simulink model "Final_Proposal"  (R2024a)
settings: Solver=ode4  StartTime=0.0  StopTime=100  FixedStep=Step_Size  RelTol=1e-3
InitFcn:
  | clc ;
  | clear all ;
  | close all ;
  | UAV_Data ;
  | Sim_Parameters ;
values from neighbouring files (symbols this model uses):
  B = 0.90    (= 0.9)    [UAV_Data.m]
  CBAR = 0.25    [UAV_Data.m]
  CD_0 = 0.0208    [UAV_Data.m]
  CD_alpha = 0.0084    [UAV_Data.m]
  CD_alpha_2 = 1.3225    [UAV_Data.m]
  CD_beta = -0.0001    [UAV_Data.m]
  CD_beta_2 = 0.0796    [UAV_Data.m]
  CD_del_e = 0.20    (= 0.2)    [UAV_Data.m]
  CD_q = 0.00    (= 0)    [UAV_Data.m]
  CL_0 = 0.0389    [UAV_Data.m]
  Cl_0 = 0.000    (= 0)    [UAV_Data.m]
  CL_alpha = 3.2684    [UAV_Data.m]
  Cl_beta = -0.0345    [UAV_Data.m]
  Cl_del_a = 0.182    [UAV_Data.m]
  CL_del_e = 0.7237    [UAV_Data.m]
  Cl_p = -0.3318    [UAV_Data.m]
  CL_q = 6.1523    [UAV_Data.m]
  Cl_r = 0.0304    [UAV_Data.m]
  Cm_0 = -0.0112    [UAV_Data.m]
  Cm_alpha = -0.2625    [UAV_Data.m]
  Cm_del_e = -0.2845    [UAV_Data.m]
  Cm_q = -1.8522    [UAV_Data.m]
  Cn_0 = 0.0000    (= 0)    [UAV_Data.m]
  Cn_beta = 0.0252    [UAV_Data.m]
  Cn_del_a = -0.0102    [UAV_Data.m]
  Cn_p = 0.002    [UAV_Data.m]
  Cn_r = -0.0192    [UAV_Data.m]
  CY_0 = 0.000    (= 0)    [UAV_Data.m]
  CY_beta = -0.1285    [UAV_Data.m]
  CY_del_a = 0.0299    [UAV_Data.m]
  CY_p = -0.0292    [UAV_Data.m]
  CY_r = -0.0355    [UAV_Data.m]
  I_TENSOR = [ I_xx,  0.0, -I_xz ... (first row only)    [UAV_Data.m]
  Init_Euler = [  0.0, 0.0, 0.0]    [Sim_Parameters.m]
  Init_Pos = [  0.0, 0.0, 0.0]    [Sim_Parameters.m]
  Init_Rate = [  0.0, 0.0, 0.0 ]    [Sim_Parameters.m]
  Init_Vel = [  12,  0.0,  0.0]    [Sim_Parameters.m]
  K_d = 0.0470    (= 0.047)    [UAV_Data.m]
  K_d_h = 0.1282    [UAV_Data.m]
  K_d_q = 0.0591    [UAV_Data.m]
  K_d_r = 0.0000    (= 0)    [UAV_Data.m]
  K_d_roll = 0.7683    [UAV_Data.m]
  K_d_theta = 0.1088    [UAV_Data.m]
  K_d_vt = 0.2171    [UAV_Data.m]
  K_I = 5.5033    [UAV_Data.m]
  K_I_h = 0.2373    [UAV_Data.m]
  K_I_q = 7.5000    (= 7.5)    [UAV_Data.m]
  K_I_r = 0.0011    [UAV_Data.m]
  K_I_roll = 0.0329    [UAV_Data.m]
  K_I_theta = 0.2536    [UAV_Data.m]
  K_I_vt = 0.0000    (= 0)    [UAV_Data.m]
  K_M = 2.444*10^(-10)    (= 2.444e-10)    [UAV_Data.m]
  K_p = 0.2631    [UAV_Data.m]
  K_p_h = 0.6879    [UAV_Data.m]
  K_p_q = 0.3    [UAV_Data.m]
  K_p_r = 1.02    [UAV_Data.m]
  K_p_roll = 22.2973    [UAV_Data.m]
  K_p_theta = 8.2978    [UAV_Data.m]
  K_p_vt = 1.4665    [UAV_Data.m]
  K_T = 2.015*10^(-6)    (= 2.015e-06)    [UAV_Data.m]
  Mass = 1    [UAV_Data.m]
  Omega_act = 9.774    [UAV_Data.m]
  tau_T = 0.19    [UAV_Data.m]
  UNIT_GRAV = 9.81    [Sim_Parameters.m]
  zeta_act = 0.801    [UAV_Data.m]
undefined symbols (not defined in the file or in its folder): deg, rad, s
libraries: aerolibconvert2 x4, simulink_extras x3, shared6dofsys x2, aerolibasang x2, sharedtransform x1, sharedutil x1, shared6dof x1, aerolibadyn x1, aerolibatmos2 x1
settings Model: Creator=Natalia C Rios  LastModifiedBy=Natalia C Rios

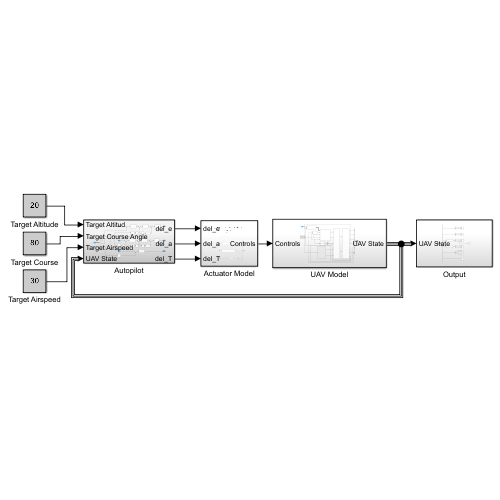
[thumbnail: Simulink's stored preview of the top-level diagram]
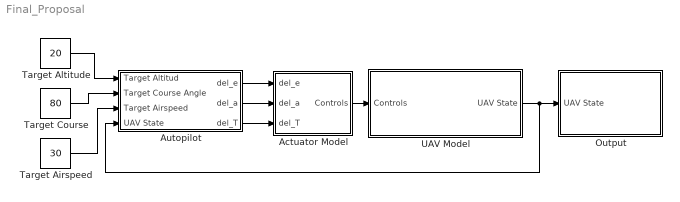
== system Final_Proposal ==
  Actuator Model : Subsystem
  Autopilot : Subsystem
  Output : Subsystem
  Target Airspeed : Constant  Value=30
  Target Altitude : Constant  Value=20
  Target Course : Constant  Value=80
  UAV Model : Subsystem
  wires:
  Target Course/1 -> Autopilot/2(Target Course Angle)
  Actuator Model/1(Controls) -> UAV Model/1(Controls)
  Autopilot/2(del_a) -> Actuator Model/2(del_a)
  Autopilot/3(del_T) -> Actuator Model/3(del_T)
  UAV Model/1(UAV State) -> Output/1(UAV State), Autopilot/4(UAV State)
  Target Airspeed/1 -> Autopilot/3("Target Airspeed ")
  Autopilot/1(del_e) -> Actuator Model/1(del_e)
  Target Altitude/1 -> Autopilot/1(Target Altitud)

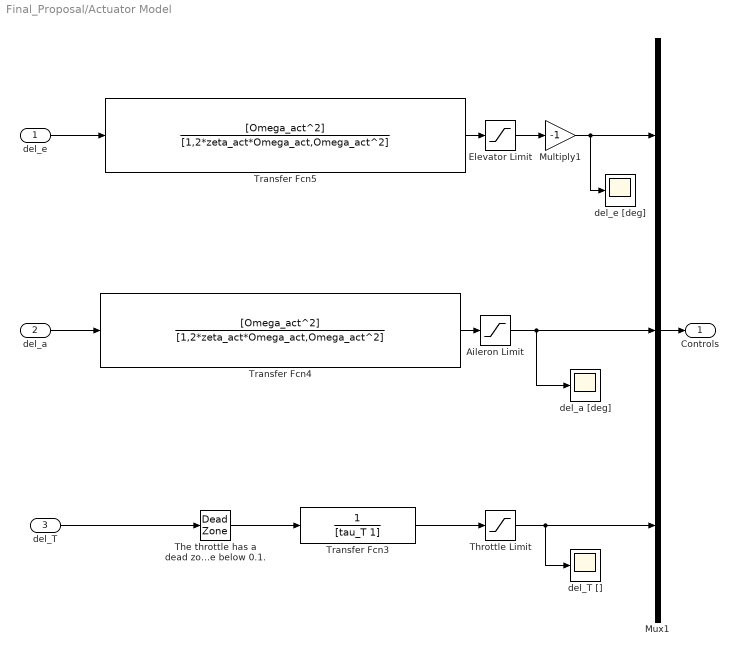
== system Final_Proposal/Actuator Model ==
  del_e : Inport
  del_a : Inport  Port=2
  del_T : Inport  Port=3
  Aileron Limit : Saturate  UpperLimit=40*pi/180  LowerLimit=-40*pi/180
  Elevator Limit : Saturate  UpperLimit=30*pi/180  LowerLimit=-30*pi/180
  Multiply1 : Gain  Gain=-1
  Mux1 : Mux  Inputs=3
  The throttle has a dead zone below 0.1. : DeadZone  LowerValue=0  UpperValue=0.1
  Throttle Limit : Saturate  UpperLimit=10  LowerLimit=0
  Transfer Fcn3 : TransferFcn  Denominator=[tau_T 1]
  Transfer Fcn4 : TransferFcn  Numerator=[Omega_act^2]  Denominator=[1,2*zeta_act*Omega_act,Omega_act^2]
  Transfer Fcn5 : TransferFcn  Numerator=[Omega_act^2]  Denominator=[1,2*zeta_act*Omega_act,Omega_act^2]
  del_T [] : Scope
  del_a [deg] : Scope
  del_e [deg] : Scope
  Controls : Outport
  wires:
  Transfer Fcn3/1 -> Throttle Limit/1
  Aileron Limit/1 -> del_a [deg]/1, Mux1/2
  Transfer Fcn4/1 -> Aileron Limit/1
  Mux1/1 -> Controls/1
  Throttle Limit/1 -> del_T []/1, Mux1/3
  del_e/1 -> Transfer Fcn5/1
  del_a/1 -> Transfer Fcn4/1
  Multiply1/1 -> del_e [deg]/1, Mux1/1
  The throttle has a dead zone below 0.1./1 -> Transfer Fcn3/1
  Elevator Limit/1 -> Multiply1/1
  del_T/1 -> The throttle has a dead zone below 0.1./1
  Transfer Fcn5/1 -> Elevator Limit/1

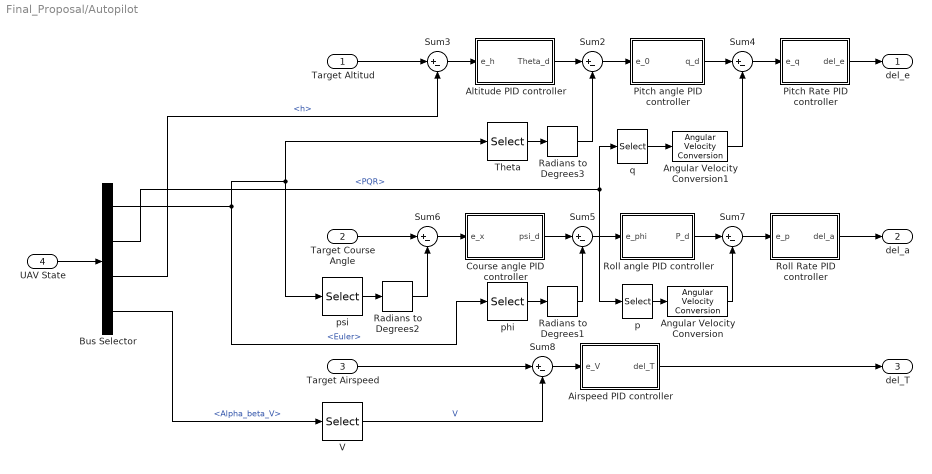
== system Final_Proposal/Autopilot ==
  Target Altitud : Inport
  Target Course Angle : Inport  Port=2
  "Target Airspeed " : Inport  Port=3
  UAV State : Inport  Port=4
  Airspeed PID controller : Subsystem
  Altitude PID controller : Subsystem
  Angular Velocity Conversion : aerolibconvert2/Angular Velocity Conversion  IU=rad/s  OU=deg/s
  Angular Velocity Conversion1 : aerolibconvert2/Angular Velocity Conversion  IU=rad/s  OU=deg/s
  Bus Selector : BusSelector  OutputSignals=Euler,PQR,h,Alpha_beta_V
  Course angle PID controller : Subsystem
  Pitch Rate PID controller : Subsystem
  Pitch angle PID controller : Subsystem
  Radians to Degrees1 : simulink_extras/Transformations/Radians to Degrees
  Radians to Degrees2 : simulink_extras/Transformations/Radians to Degrees
  Radians to Degrees3 : simulink_extras/Transformations/Radians to Degrees
  Roll Rate PID controller : Subsystem
  Roll angle PID controller : Subsystem
  Sum{2..8} (7 alike) : Sum  Inputs=|+-
  Theta : Selector  InputPortWidth=3  IndexOptions=Index vector (dialog)  Indices=[2]  OutputSizes=1
  V : Selector  InputPortWidth=3  IndexOptions=Index vector (dialog)  Indices=[3]  OutputSizes=1
  p : Selector  InputPortWidth=3  IndexOptions=Index vector (dialog)  Indices=[1]  OutputSizes=1
  phi : Selector  InputPortWidth=3  IndexOptions=Index vector (dialog)  Indices=[1]  OutputSizes=1
  psi : Selector  InputPortWidth=3  IndexOptions=Index vector (dialog)  Indices=[3]  OutputSizes=1
  q : Selector  InputPortWidth=3  IndexOptions=Index vector (dialog)  Indices=[2]  OutputSizes=1
  del_e : Outport
  del_a : Outport  Port=2
  del_T : Outport  Port=3
  wires:
  Bus Selector/3 -> Sum3/2  "<h>"
  phi/1 -> Radians to Degrees1/1
  Bus Selector/2 -> p/1, q/1  "<PQR>"
  Angular Velocity Conversion1/1 -> Sum4/2
  Sum7/1 -> Roll Rate PID controller/1(e_p)
  Pitch angle PID controller/1(q_d) -> Sum4/1
  Radians to Degrees2/1 -> Sum6/2
  Radians to Degrees3/1 -> Sum2/2
  Radians to Degrees1/1 -> Sum5/2
  Sum6/1 -> Course angle PID controller/1(e_x)
  q/1 -> Angular Velocity Conversion1/1
  p/1 -> Angular Velocity Conversion/1
  Roll Rate PID controller/1(del_a) -> del_a/1
  Airspeed PID controller/1(del_T) -> del_T/1
  Sum5/1 -> Roll angle PID controller/1(e_phi)
  Sum4/1 -> Pitch Rate PID controller/1(e_q)
  V/1 -> Sum8/2  "V"
  Sum2/1 -> Pitch angle PID controller/1(e_0)
  Course angle PID controller/1(psi_d) -> Sum5/1
  Angular Velocity Conversion/1 -> Sum7/2
  Sum8/1 -> Airspeed PID controller/1(e_V)
  Bus Selector/1 -> psi/1, Theta/1, phi/1  "<Euler>"
  psi/1 -> Radians to Degrees2/1
  Theta/1 -> Radians to Degrees3/1
  Roll angle PID controller/1(P_d) -> Sum7/1
  Target Course Angle/1 -> Sum6/1
  UAV State/1 -> Bus Selector/1
  Altitude PID controller/1(Theta_d) -> Sum2/1
  Pitch Rate PID controller/1(del_e) -> del_e/1
  "Target Airspeed "/1 -> Sum8/1
  Target Altitud/1 -> Sum3/1
  Sum3/1 -> Altitude PID controller/1(e_h)
  Bus Selector/4 -> V/1  "<Alpha_beta_V>"

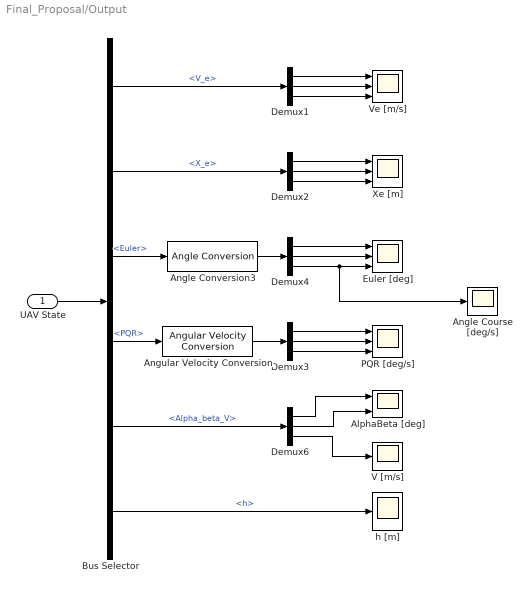
== system Final_Proposal/Output ==
  UAV State : Inport
  AlphaBeta [deg] : Scope  NumInputPorts=2
  Angle Conversion3 : aerolibconvert2/Angle Conversion  IU=rad  OU=deg
  Angle Course [deg/s] : Scope
  Angular Velocity Conversion : aerolibconvert2/Angular Velocity Conversion  IU=rad/s  OU=deg/s
  Bus Selector : BusSelector  OutputSignals=V_e,X_e,Euler,PQR,Alpha_beta_V,h
  Demux{1..4,6} (5 alike) : Demux  Outputs=3
  Euler [deg] : Scope  NumInputPorts=3
  PQR [deg/s] : Scope  NumInputPorts=3
  V [m/s] : Scope
  Ve [m/s] : Scope  NumInputPorts=3
  Xe [m] : Scope  NumInputPorts=3
  h [m] : Scope
  wires:
  Demux1/3 -> Ve [m/s]/3
  Demux6/1 -> AlphaBeta [deg]/1
  Demux4/3 -> Angle Course [deg/s]/1, Euler [deg]/3
  Demux3/1 -> PQR [deg/s]/1
  Demux3/3 -> PQR [deg/s]/3
  Demux4/2 -> Euler [deg]/2
  Demux2/3 -> Xe [m]/3
  Demux4/1 -> Euler [deg]/1
  Bus Selector/2 -> Demux2/1  "<X_e>"
  Bus Selector/3 -> Angle Conversion3/1  "<Euler>"
  Bus Selector/1 -> Demux1/1  "<V_e>"
  Angle Conversion3/1 -> Demux4/1
  Demux1/2 -> Ve [m/s]/2
  Demux2/2 -> Xe [m]/2
  UAV State/1 -> Bus Selector/1
  Demux2/1 -> Xe [m]/1
  Demux6/2 -> AlphaBeta [deg]/2
  Bus Selector/4 -> Angular Velocity Conversion/1  "<PQR>"
  Demux1/1 -> Ve [m/s]/1
  Bus Selector/6 -> h [m]/1  "<h>"
  Demux3/2 -> PQR [deg/s]/2
  Angular Velocity Conversion/1 -> Demux3/1
  Demux6/3 -> V [m/s]/1
  Bus Selector/5 -> Demux6/1  "<Alpha_beta_V>"

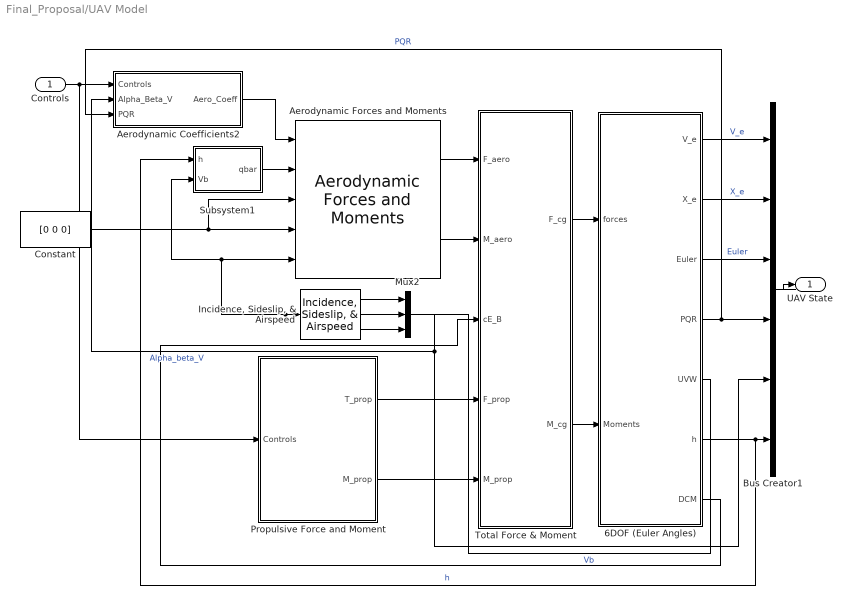
== system Final_Proposal/UAV Model ==
  Controls : Inport
  6DOF (Euler Angles) : Subsystem
  "Aerodynamic Forces and Moments " : aerolibadyn/Aerodynamic Forces and Moments   inputAxes=Stability  outputForceAxes=Body  outputMomentAxes=Body  S=S  b=B  cbar=CBAR
  Aerodynamic Coefficients2 : Subsystem
  Bus Creator1 : BusCreator  Inputs=6
  Constant : Constant  Value=[0 0 0]
  "Incidence, Sideslip, & Airspeed" : aerolibasang/Incidence, Sideslip, & Airspeed
  Mux2 : Mux  Inputs=3
  Propulsive Force and Moment : Subsystem
  Subsystem1 : Subsystem
  Total Force & Moment : Subsystem
  UAV State : Outport
  wires:
  6DOF (Euler Angles)/7(DCM) -> Total Force & Moment/3(cE_B)
  Total Force & Moment/2(M_cg) -> 6DOF (Euler Angles)/2(Moments)
  Propulsive Force and Moment/1(T_prop) -> Total Force & Moment/4(F_prop)
  Constant/1 -> "Aerodynamic Forces and Moments "/3, "Aerodynamic Forces and Moments "/4
  Total Force & Moment/1(F_cg) -> 6DOF (Euler Angles)/1(forces)
  Propulsive Force and Moment/2(M_prop) -> Total Force & Moment/5(M_prop)
  Aerodynamic Coefficients2/1(Aero_Coeff) -> "Aerodynamic Forces and Moments "/1
  Subsystem1/1(qbar) -> "Aerodynamic Forces and Moments "/2
  Controls/1 -> Propulsive Force and Moment/1(Controls), Aerodynamic Coefficients2/1(Controls)
  "Incidence, Sideslip, & Airspeed"/3 -> Mux2/3
  "Incidence, Sideslip, & Airspeed"/2 -> Mux2/2
  "Incidence, Sideslip, & Airspeed"/1 -> Mux2/1
  Mux2/1 -> Bus Creator1/5, Aerodynamic Coefficients2/2(Alpha_Beta_V)  "Alpha_beta_V"
  Bus Creator1/1 -> UAV State/1
  6DOF (Euler Angles)/1(V_e) -> Bus Creator1/1  "V_e"
  6DOF (Euler Angles)/5(UVW) -> "Aerodynamic Forces and Moments "/5, Subsystem1/2(Vb), "Incidence, Sideslip, & Airspeed"/1  "Vb"
  6DOF (Euler Angles)/4(PQR) -> Bus Creator1/4, Aerodynamic Coefficients2/3(PQR)  "PQR"
  6DOF (Euler Angles)/2(X_e) -> Bus Creator1/2  "X_e"
  6DOF (Euler Angles)/3(Euler) -> Bus Creator1/3  "Euler"
  6DOF (Euler Angles)/6(h) -> Subsystem1/1(h), Bus Creator1/6  "h"
  "Aerodynamic Forces and Moments "/1 -> Total Force & Moment/1(F_aero)
  "Aerodynamic Forces and Moments "/2 -> Total Force & Moment/2(M_aero)

== system Final_Proposal/Autopilot/Airspeed PID controller ==
  e_V : Inport
  Derivative : Derivative
  Integrator : Integrator
  Kd : Gain  Gain=K_d_vt
  Ki : Gain  Gain=K_I_vt
  Kp : Gain  Gain=K_p_vt
  Sum : Sum  Inputs=+++
  del_T : Outport
  wires:
  Derivative/1 -> Sum/3
  e_V/1 -> Kd/1, Ki/1, Kp/1
  Kd/1 -> Derivative/1
  Ki/1 -> Integrator/1
  Integrator/1 -> Sum/2
  Kp/1 -> Sum/1
  Sum/1 -> del_T/1

== system Final_Proposal/Autopilot/Altitude PID controller ==
  e_h : Inport
  Derivative : Derivative
  Integrator : Integrator
  Kd : Gain  Gain=K_d_h
  Ki : Gain  Gain=K_I_h
  Kp : Gain  Gain=K_p_h
  Sum : Sum  Inputs=+++
  Theta_d : Outport
  wires:
  Sum/1 -> Theta_d/1
  Derivative/1 -> Sum/3
  Ki/1 -> Integrator/1
  e_h/1 -> Kd/1, Ki/1, Kp/1
  Kd/1 -> Derivative/1
  Kp/1 -> Sum/1
  Integrator/1 -> Sum/2

== system Final_Proposal/Autopilot/Course angle PID controller ==
  e_x : Inport
  Derivative : Derivative
  Integrator : Integrator
  Kd : Gain  Gain=K_d_r
  Ki : Gain  Gain=K_I_r
  Kp : Gain  Gain=K_p_r*0.2
  Sum : Sum  Inputs=+++
  psi_d : Outport
  wires:
  Sum/1 -> psi_d/1
  Derivative/1 -> Sum/3
  Ki/1 -> Integrator/1
  e_x/1 -> Kd/1, Ki/1, Kp/1
  Kd/1 -> Derivative/1
  Kp/1 -> Sum/1
  Integrator/1 -> Sum/2

== system Final_Proposal/Autopilot/Pitch Rate PID controller ==
  e_q : Inport
  Derivative : Derivative
  Integrator : Integrator
  Kd : Gain  Gain=K_d_q
  Ki : Gain  Gain=K_I_q
  Kp : Gain  Gain=K_p_q
  Sum : Sum  Inputs=+++
  del_e : Outport
  wires:
  Sum/1 -> del_e/1
  Derivative/1 -> Sum/3
  Ki/1 -> Integrator/1
  e_q/1 -> Kd/1, Ki/1, Kp/1
  Kd/1 -> Derivative/1
  Kp/1 -> Sum/1
  Integrator/1 -> Sum/2

== system Final_Proposal/Autopilot/Pitch angle PID controller ==
  e_0 : Inport
  Derivative : Derivative
  Integrator : Integrator
  Kd : Gain  Gain=K_d_theta
  Ki : Gain  Gain=K_I_theta
  Kp : Gain  Gain=K_p_theta
  Sum : Sum  Inputs=+++
  q_d : Outport
  wires:
  Sum/1 -> q_d/1
  Derivative/1 -> Sum/3
  Ki/1 -> Integrator/1
  e_0/1 -> Kd/1, Ki/1, Kp/1
  Kd/1 -> Derivative/1
  Kp/1 -> Sum/1
  Integrator/1 -> Sum/2

== system Final_Proposal/Autopilot/Roll Rate PID controller ==
  e_p : Inport
  Derivative : Derivative
  Integrator : Integrator
  Kd : Gain  Gain=K_d
  Ki : Gain  Gain=K_I
  Kp : Gain  Gain=K_p
  Sum : Sum  Inputs=+++
  del_a : Outport
  wires:
  Sum/1 -> del_a/1
  Derivative/1 -> Sum/3
  Ki/1 -> Integrator/1
  e_p/1 -> Kd/1, Ki/1, Kp/1
  Kd/1 -> Derivative/1
  Kp/1 -> Sum/1
  Integrator/1 -> Sum/2

== system Final_Proposal/Autopilot/Roll angle PID controller ==
  e_phi : Inport
  Derivative : Derivative
  Integrator : Integrator
  Kd : Gain  Gain=K_d_roll
  Ki : Gain  Gain=K_I_roll
  Kp : Gain  Gain=K_p_roll
  Sum : Sum  Inputs=+++
  P_d : Outport
  wires:
  Sum/1 -> P_d/1
  Derivative/1 -> Sum/3
  Ki/1 -> Integrator/1
  e_phi/1 -> Kd/1, Ki/1, Kp/1
  Kd/1 -> Derivative/1
  Kp/1 -> Sum/1
  Integrator/1 -> Sum/2

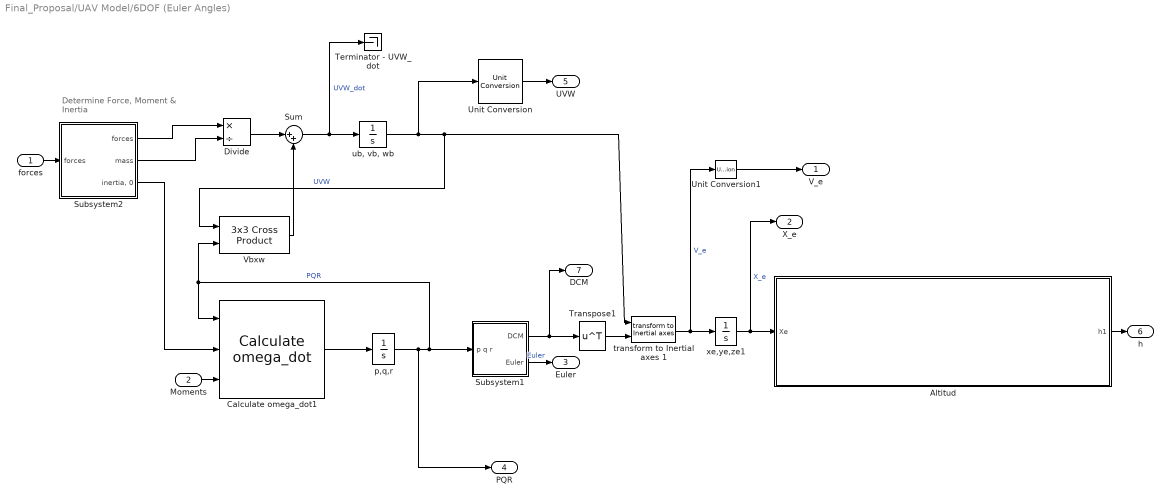
== system Final_Proposal/UAV Model/6DOF (Euler Angles) ==
  note: Determine Force, Moment & Inertia
  forces : Inport
  Moments : Inport  Port=2
  Altitud : Subsystem
  Calculate omega_dot1 : shared6dofsys/Calculate omega_dot  aMode=aMode
  Divide : Product  Inputs=*/
  Subsystem1 : Subsystem
  Subsystem2 : Subsystem
  Sum : Sum  Inputs=|++
  Terminator - UVW_dot : Terminator
  Transpose1 : Math  Operator=transpose
  Unit Conversion : UnitConversion
  Unit Conversion1 : UnitConversion
  Vbxw : sharedutil/3x3 Cross Product  aMode=aMode
  p,q,r : Integrator  InitialCondition=Init_Rate
  transform to Inertial axes 1 : shared6dof/6DOF (Euler Angles)/transform to Inertial axes   SystemSampleTime=-1  VariantActivationTime=update diagram  AllowFlexibleInterface=on  Latency=0  AutoFrameSizeCalculation=off
  "ub, vb, wb" : Integrator  InitialCondition=Init_Vel
  xe,ye,ze1 : Integrator  InitialCondition=Init_Pos
  V_e : Outport
  X_e : Outport  Port=2
  Euler : Outport  Port=3
  PQR : Outport  Port=4
  UVW : Outport  Port=5
  h : Outport  Port=6
  DCM : Outport  Port=7
  wires:
  Divide/1 -> Sum/1
  transform to Inertial axes 1/1 -> Unit Conversion1/1, xe,ye,ze1/1  "V_e"
  Transpose1/1 -> transform to Inertial axes 1/2
  xe,ye,ze1/1 -> X_e/1, Altitud/1(Xe)  "X_e"
  Vbxw/1 -> Sum/2
  Sum/1 -> "ub, vb, wb"/1, Terminator - UVW_dot/1  "UVW_dot"
  Subsystem2/1("forces ") -> Divide/1
  Altitud/1(h1) -> h/1
  Subsystem2/3("inertia, 0") -> Calculate omega_dot1/2
  p,q,r/1 -> PQR/1, Vbxw/2, Calculate omega_dot1/1, Subsystem1/1("p q r ")  "PQR"
  Calculate omega_dot1/1 -> p,q,r/1
  "ub, vb, wb"/1 -> Unit Conversion/1, Vbxw/1, transform to Inertial axes 1/1  "UVW"
  Subsystem1/1(DCM) -> DCM/1, Transpose1/1
  Moments/1 -> Calculate omega_dot1/3
  Subsystem2/2(mass) -> Divide/2
  forces/1 -> Subsystem2/1(forces)
  Subsystem1/2(Euler) -> Euler/1  "Euler"
  Unit Conversion/1 -> UVW/1
  Unit Conversion1/1 -> V_e/1

== system Final_Proposal/UAV Model/Aerodynamic Coefficients2 ==
  note: Lift Force Coefficient
  note: Side Force Coefficient
  note: Drag Force Coefficient
  note: Rolling Moment Coefficient
  note: Pitching Moment Coefficient
  note: Yawing Moment Coefficient
  Controls : Inport
  Alpha_Beta_V : Inport  Port=2
  PQR : Inport  Port=3
  Bus Creator : BusCreator  Inputs=6
  Drag Force Coefficient : Subsystem
  Lift Force Coefficient : Subsystem
  Pitching Moment Coefficient : Subsystem
  Rolling Moment Coefficient : Subsystem
  Side Force Coefficient : Subsystem
  Yawing Moment Coefficient1 : Subsystem
  Aero_Coeff : Outport
  wires:
  Alpha_Beta_V/1 -> Lift Force Coefficient/2(Alpha_Beta_V), Yawing Moment Coefficient1/1(Alpha_Beta_V), Rolling Moment Coefficient/1(Alpha_Beta_V), Pitching Moment Coefficient/2(Alpha_Beta_V), Side Force Coefficient/1(Alpha_Beta_V), Drag Force Coefficient/2(Alpha_Beta_V)
  Controls/1 -> Lift Force Coefficient/1(Controls), Side Force Coefficient/3(Controls), Yawing Moment Coefficient1/3(Controls), Rolling Moment Coefficient/3(Controls), Pitching Moment Coefficient/1(Controls), Drag Force Coefficient/1(Controls)
  Bus Creator/1 -> Aero_Coeff/1
  PQR/1 -> Lift Force Coefficient/3(PQR_s), Yawing Moment Coefficient1/2(PQR_s), Rolling Moment Coefficient/2(PQR_s), Pitching Moment Coefficient/3(PQR_s), Side Force Coefficient/2(PQR_s), Drag Force Coefficient/3(PQR_s)
  Drag Force Coefficient/1(CD) -> Bus Creator/1  "CD"
  Side Force Coefficient/1(CY) -> Bus Creator/2  "CY"
  Lift Force Coefficient/1(CL) -> Bus Creator/3  "CL"
  Pitching Moment Coefficient/1(Cm) -> Bus Creator/5  "Cm"
  Rolling Moment Coefficient/1(Cl) -> Bus Creator/4  "Cl"
  Yawing Moment Coefficient1/1(Cn) -> Bus Creator/6  "Cn"

== system Final_Proposal/UAV Model/Propulsive Force and Moment ==
  Controls : Inport
  Constant : Constant  Value=0
  Constant2 : Constant  Value=0
  Gain : Gain  Gain=K_T
  Gain1 : Gain  Gain=K_M
  Mux : Mux  Inputs=3
  Mux1 : Mux  Inputs=3
  N(RPS) : Subsystem
  Square : Math  Operator=square
  T_prop : Outport  VectorParamsAs1DForOutWhenUnconnected=off
  M_prop : Outport  Port=2  VectorParamsAs1DForOutWhenUnconnected=off
  wires:
  Square/1 -> Gain/1, Gain1/1
  Constant/1 -> Mux/2, Mux/3
  Constant2/1 -> Mux1/2, Mux1/3
  Gain1/1 -> Mux1/1
  Gain/1 -> Mux/1
  Mux/1 -> T_prop/1
  Mux1/1 -> M_prop/1
  Controls/1 -> N(RPS)/1(Controls)
  N(RPS)/1(Out1) -> Square/1

== system Final_Proposal/UAV Model/Subsystem1 ==
  h : Inport
  Vb : Inport  Port=2
  Altitude - ISA Analysis : Subsystem
  Dynamic Pressure : aerolibasang/Dynamic Pressure
  qbar : Outport
  wires:
  Altitude - ISA Analysis/1(Rho) -> Dynamic Pressure/2
  h/1 -> Altitude - ISA Analysis/1(h)
  Dynamic Pressure/1 -> qbar/1
  Vb/1 -> Dynamic Pressure/1

== system Final_Proposal/UAV Model/Total Force & Moment ==
  F_aero : Inport
  M_aero : Inport  Port=2
  cE_B : Inport  Port=3
  F_prop : Inport  Port=4
  M_prop : Inport  Port=5
  Subsystem : Subsystem
  Total Force & Moment : Subsystem  AncestorBlock=UAS_Model_library/External Forces/Total Force & Moment
  F_cg : Outport
  M_cg : Outport  Port=2
  wires:
  M_prop/1 -> Total Force & Moment/5(M_prop)
  M_aero/1 -> Total Force & Moment/2(M_aero)
  Subsystem/1(Gravity) -> Total Force & Moment/3(F_gravity)
  F_aero/1 -> Total Force & Moment/1(F_aero)
  F_prop/1 -> Total Force & Moment/4(F_prop)
  Total Force & Moment/2(M_cg) -> M_cg/1
  cE_B/1 -> Subsystem/1(cE_B)
  Total Force & Moment/1(F_cg) -> F_cg/1

== system Final_Proposal/UAV Model/6DOF (Euler Angles)/Altitud ==
  Xe : Inport
  Z_e : Selector  InputPortWidth=3  IndexOptions=Index vector (dialog)  Indices=[3]  OutputSizes=1
  conv : Gain  Gain=-1
  h1 : Outport  VectorParamsAs1DForOutWhenUnconnected=off
  wires:
  Z_e/1 -> conv/1
  Xe/1 -> Z_e/1
  conv/1 -> h1/1

== system Final_Proposal/UAV Model/6DOF (Euler Angles)/Subsystem1 ==
  "p q r " : Inport
  Rotation Angles to Direction Cosine Matrix : sharedtransform/Rotation Angles to Direction Cosine Matrix  rotationOrder=ZYX  aMode=aMode
  Selector : Selector  InputPortWidth=3  IndexOptions=Index vector (dialog)  Indices=[3 2 1]  OutputSizes=1
  phi theta psi : Integrator  InitialCondition=Init_Euler
  phidot thetadot psidot : shared6dofsys/DCM & Euler Angles (Euler)/phidot thetadot psidot  SystemSampleTime=-1  VariantActivationTime=update diagram  AllowFlexibleInterface=on  Latency=0  AutoFrameSizeCalculation=off
  DCM : Outport  VectorParamsAs1DForOutWhenUnconnected=off
  Euler : Outport  Port=2  VectorParamsAs1DForOutWhenUnconnected=off
  wires:
  phi theta psi/1 -> Euler/1, Selector/1, phidot thetadot psidot/2
  Rotation Angles to Direction Cosine Matrix/1 -> DCM/1
  Selector/1 -> Rotation Angles to Direction Cosine Matrix/1
  "p q r "/1 -> phidot thetadot psidot/1
  phidot thetadot psidot/1 -> phi theta psi/1

== system Final_Proposal/UAV Model/6DOF (Euler Angles)/Subsystem2 ==
  forces : Inport
  Constant : Constant  Value=Mass  OutDataTypeStr=Inherit: Inherit via back propagation
  Constant1 : Constant  Value=I_TENSOR  OutDataTypeStr=Inherit: Inherit via back propagation
  Constant2 : Constant  Value=zeros(3)
  Vector Concatenate : Concatenate  Mode=Multidimensional array
  "forces " : Outport  VectorParamsAs1DForOutWhenUnconnected=off
  mass : Outport  Port=2  VectorParamsAs1DForOutWhenUnconnected=off
  "inertia, 0" : Outport  Port=3  VectorParamsAs1DForOutWhenUnconnected=off
  wires:
  Constant/1 -> mass/1
  Constant2/1 -> Vector Concatenate/2
  forces/1 -> "forces "/1
  Constant1/1 -> Vector Concatenate/1
  Vector Concatenate/1 -> "inertia, 0"/1

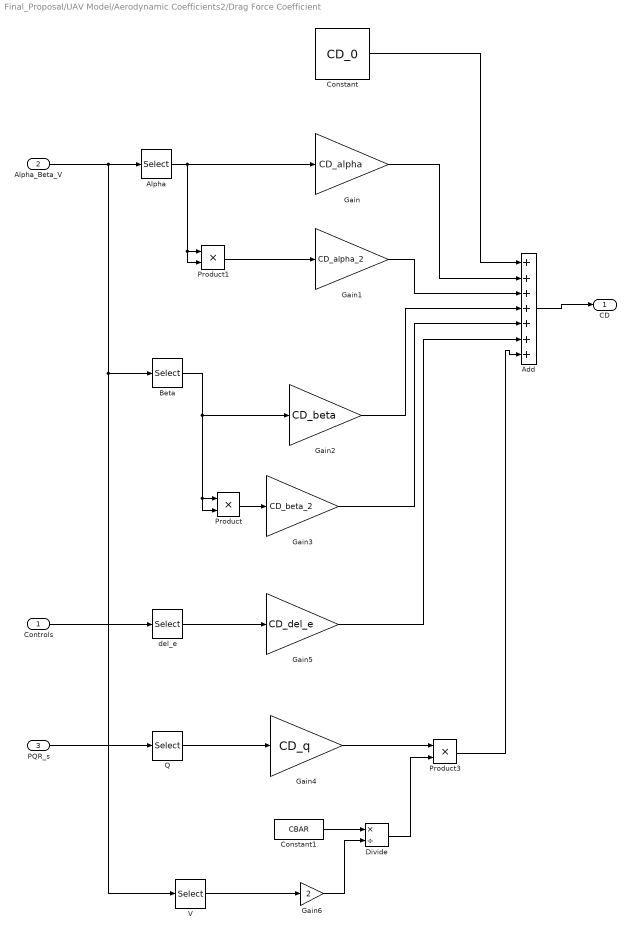
== system Final_Proposal/UAV Model/Aerodynamic Coefficients2/Drag Force Coefficient ==
  Controls : Inport
  Alpha_Beta_V : Inport  Port=2
  PQR_s : Inport  Port=3
  Add : Sum  Inputs=+++++++
  Alpha : Selector  InputPortWidth=3  IndexOptions=Index vector (dialog)  Indices=[1]  OutputSizes=1
  Beta : Selector  InputPortWidth=3  IndexOptions=Index vector (dialog)  Indices=[2]  OutputSizes=1
  Constant : Constant  Value=CD_0
  Constant1 : Constant  Value=CBAR
  Divide : Product  Inputs=*/
  Gain : Gain  Gain=CD_alpha
  Gain1 : Gain  Gain=CD_alpha_2
  Gain2 : Gain  Gain=CD_beta
  Gain3 : Gain  Gain=CD_beta_2
  Gain4 : Gain  Gain=CD_q
  Gain5 : Gain  Gain=CD_del_e
  Gain6 : Gain  Gain=2
  Product : Product
  Product1 : Product
  Product3 : Product
  Q : Selector  InputPortWidth=3  IndexOptions=Index vector (dialog)  Indices=[2]  OutputSizes=1
  V : Selector  InputPortWidth=3  IndexOptions=Index vector (dialog)  Indices=[3]  OutputSizes=1
  del_e : Selector  InputPortWidth=3  IndexOptions=Index vector (dialog)  Indices=[1]  OutputSizes=1
  CD : Outport  VectorParamsAs1DForOutWhenUnconnected=off
  wires:
  Alpha/1 -> Product1/2, Product1/1, Gain/1
  Alpha_Beta_V/1 -> V/1, Beta/1, Alpha/1
  Beta/1 -> Product/2, Product/1, Gain2/1
  del_e/1 -> Gain5/1
  Controls/1 -> del_e/1
  V/1 -> Gain6/1
  Constant1/1 -> Divide/1
  Gain6/1 -> Divide/2
  Gain4/1 -> Product3/1
  Divide/1 -> Product3/2
  PQR_s/1 -> Q/1
  Q/1 -> Gain4/1
  Gain/1 -> Add/2
  Constant/1 -> Add/1
  Gain1/1 -> Add/3
  Gain2/1 -> Add/4
  Gain3/1 -> Add/5
  Gain5/1 -> Add/6
  Product1/1 -> Gain1/1
  Product/1 -> Gain3/1
  Add/1 -> CD/1
  Product3/1 -> Add/7

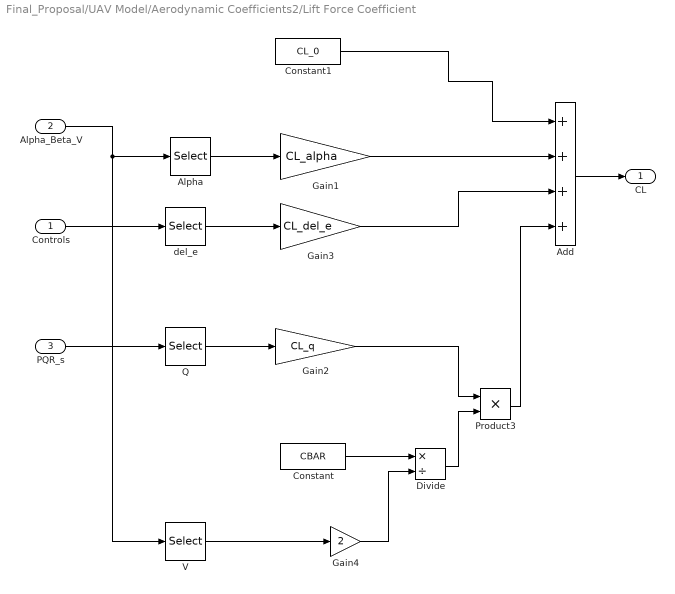
== system Final_Proposal/UAV Model/Aerodynamic Coefficients2/Lift Force Coefficient ==
  Controls : Inport
  Alpha_Beta_V : Inport  Port=2
  PQR_s : Inport  Port=3
  Add : Sum  Inputs=++++
  Alpha : Selector  InputPortWidth=3  IndexOptions=Index vector (dialog)  Indices=[1]  OutputSizes=1
  Constant : Constant  Value=CBAR
  Constant1 : Constant  Value=CL_0
  Divide : Product  Inputs=*/
  Gain1 : Gain  Gain=CL_alpha
  Gain2 : Gain  Gain=CL_q
  Gain3 : Gain  Gain=CL_del_e
  Gain4 : Gain  Gain=2
  Product3 : Product
  Q : Selector  InputPortWidth=3  IndexOptions=Index vector (dialog)  Indices=[2]  OutputSizes=1
  V : Selector  InputPortWidth=3  IndexOptions=Index vector (dialog)  Indices=[3]  OutputSizes=1
  del_e : Selector  InputPortWidth=3  IndexOptions=Index vector (dialog)  Indices=[1]  OutputSizes=1
  CL : Outport  VectorParamsAs1DForOutWhenUnconnected=off
  wires:
  Gain4/1 -> Divide/2
  V/1 -> Gain4/1
  Constant/1 -> Divide/1
  Divide/1 -> Product3/2
  Gain2/1 -> Product3/1
  Q/1 -> Gain2/1
  Alpha/1 -> Gain1/1
  del_e/1 -> Gain3/1
  Controls/1 -> del_e/1
  Alpha_Beta_V/1 -> V/1, Alpha/1
  PQR_s/1 -> Q/1
  Product3/1 -> Add/4
  Gain3/1 -> Add/3
  Gain1/1 -> Add/2
  Constant1/1 -> Add/1
  Add/1 -> CL/1

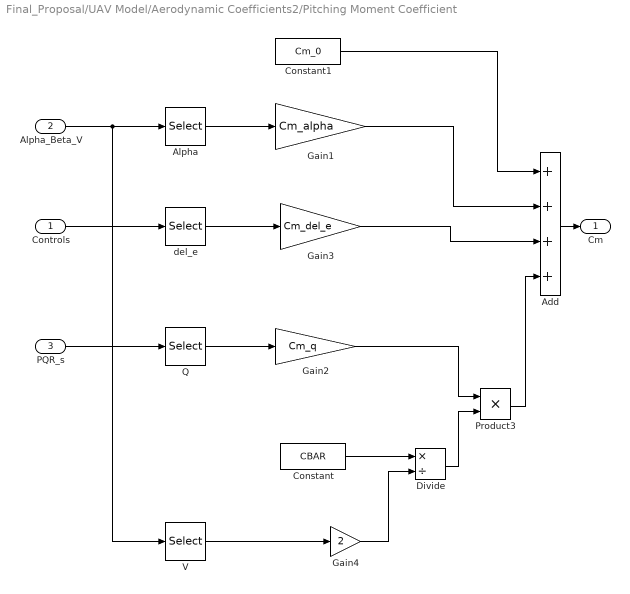
== system Final_Proposal/UAV Model/Aerodynamic Coefficients2/Pitching Moment Coefficient ==
  Controls : Inport
  Alpha_Beta_V : Inport  Port=2
  PQR_s : Inport  Port=3
  Add : Sum  Inputs=++++
  Alpha : Selector  InputPortWidth=3  IndexOptions=Index vector (dialog)  Indices=[1]  OutputSizes=1
  Constant : Constant  Value=CBAR
  Constant1 : Constant  Value=Cm_0
  Divide : Product  Inputs=*/
  Gain1 : Gain  Gain=Cm_alpha
  Gain2 : Gain  Gain=Cm_q
  Gain3 : Gain  Gain=Cm_del_e
  Gain4 : Gain  Gain=2
  Product3 : Product
  Q : Selector  InputPortWidth=3  IndexOptions=Index vector (dialog)  Indices=[2]  OutputSizes=1
  V : Selector  InputPortWidth=3  IndexOptions=Index vector (dialog)  Indices=[3]  OutputSizes=1
  del_e : Selector  InputPortWidth=3  IndexOptions=Index vector (dialog)  Indices=[1]  OutputSizes=1
  Cm : Outport  VectorParamsAs1DForOutWhenUnconnected=off
  wires:
  Q/1 -> Gain2/1
  Gain2/1 -> Product3/1
  Controls/1 -> del_e/1
  del_e/1 -> Gain3/1
  Gain3/1 -> Add/3
  Product3/1 -> Add/4
  Alpha/1 -> Gain1/1
  Constant1/1 -> Add/1
  Gain1/1 -> Add/2
  PQR_s/1 -> Q/1
  Divide/1 -> Product3/2
  Gain4/1 -> Divide/2
  Alpha_Beta_V/1 -> V/1, Alpha/1
  V/1 -> Gain4/1
  Constant/1 -> Divide/1
  Add/1 -> Cm/1

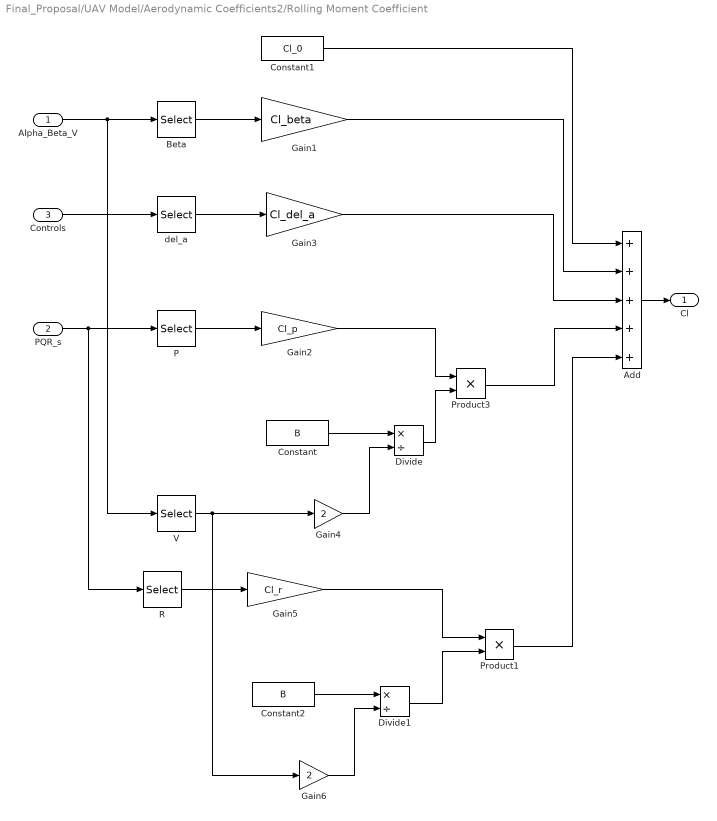
== system Final_Proposal/UAV Model/Aerodynamic Coefficients2/Rolling Moment Coefficient ==
  Alpha_Beta_V : Inport
  PQR_s : Inport  Port=2
  Controls : Inport  Port=3
  Add : Sum  Inputs=+++++
  Beta : Selector  InputPortWidth=3  IndexOptions=Index vector (dialog)  Indices=[2]  OutputSizes=1
  Constant : Constant  Value=B
  Constant1 : Constant  Value=Cl_0
  Constant2 : Constant  Value=B
  Divide : Product  Inputs=*/
  Divide1 : Product  Inputs=*/
  Gain1 : Gain  Gain=Cl_beta
  Gain2 : Gain  Gain=Cl_p
  Gain3 : Gain  Gain=Cl_del_a
  Gain4 : Gain  Gain=2
  Gain5 : Gain  Gain=Cl_r
  Gain6 : Gain  Gain=2
  P : Selector  InputPortWidth=3  IndexOptions=Index vector (dialog)  Indices=[1]  OutputSizes=1
  Product1 : Product
  Product3 : Product
  R : Selector  InputPortWidth=3  IndexOptions=Index vector (dialog)  Indices=[3]  OutputSizes=1
  V : Selector  InputPortWidth=3  IndexOptions=Index vector (dialog)  Indices=[3]  OutputSizes=1
  del_a : Selector  InputPortWidth=3  IndexOptions=Index vector (dialog)  Indices=[2]  OutputSizes=1
  Cl : Outport  VectorParamsAs1DForOutWhenUnconnected=off
  wires:
  R/1 -> Gain5/1
  Divide1/1 -> Product1/2
  Constant2/1 -> Divide1/1
  Gain6/1 -> Divide1/2
  Gain5/1 -> Product1/1
  V/1 -> Gain6/1, Gain4/1
  Gain1/1 -> Add/2
  Constant/1 -> Divide/1
  PQR_s/1 -> R/1, P/1
  Gain4/1 -> Divide/2
  Gain3/1 -> Add/3
  Divide/1 -> Product3/2
  Gain2/1 -> Product3/1
  Constant1/1 -> Add/1
  Alpha_Beta_V/1 -> V/1, Beta/1
  Beta/1 -> Gain1/1
  P/1 -> Gain2/1
  Product3/1 -> Add/4
  Product1/1 -> Add/5
  del_a/1 -> Gain3/1
  Controls/1 -> del_a/1
  Add/1 -> Cl/1

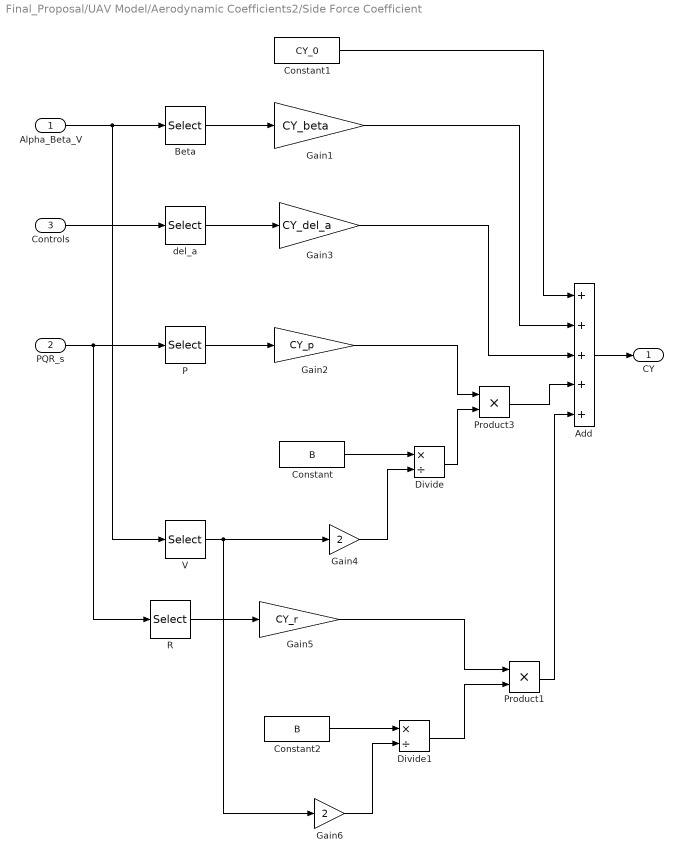
== system Final_Proposal/UAV Model/Aerodynamic Coefficients2/Side Force Coefficient ==
  Alpha_Beta_V : Inport
  PQR_s : Inport  Port=2
  Controls : Inport  Port=3
  Add : Sum  Inputs=+++++
  Beta : Selector  InputPortWidth=3  IndexOptions=Index vector (dialog)  Indices=[2]  OutputSizes=1
  Constant : Constant  Value=B
  Constant1 : Constant  Value=CY_0
  Constant2 : Constant  Value=B
  Divide : Product  Inputs=*/
  Divide1 : Product  Inputs=*/
  Gain1 : Gain  Gain=CY_beta
  Gain2 : Gain  Gain=CY_p
  Gain3 : Gain  Gain=CY_del_a
  Gain4 : Gain  Gain=2
  Gain5 : Gain  Gain=CY_r
  Gain6 : Gain  Gain=2
  P : Selector  InputPortWidth=3  IndexOptions=Index vector (dialog)  Indices=[1]  OutputSizes=1
  Product1 : Product
  Product3 : Product
  R : Selector  InputPortWidth=3  IndexOptions=Index vector (dialog)  Indices=[3]  OutputSizes=1
  V : Selector  InputPortWidth=3  IndexOptions=Index vector (dialog)  Indices=[3]  OutputSizes=1
  del_a : Selector  InputPortWidth=3  IndexOptions=Index vector (dialog)  Indices=[2]  OutputSizes=1
  CY : Outport  VectorParamsAs1DForOutWhenUnconnected=off
  wires:
  P/1 -> Gain2/1
  Gain2/1 -> Product3/1
  Gain3/1 -> Add/3
  Beta/1 -> Gain1/1
  Constant1/1 -> Add/1
  Gain1/1 -> Add/2
  Divide/1 -> Product3/2
  Gain4/1 -> Divide/2
  V/1 -> Gain6/1, Gain4/1
  Constant/1 -> Divide/1
  Controls/1 -> del_a/1
  del_a/1 -> Gain3/1
  Gain6/1 -> Divide1/2
  Divide1/1 -> Product1/2
  Gain5/1 -> Product1/1
  PQR_s/1 -> R/1, P/1
  Constant2/1 -> Divide1/1
  R/1 -> Gain5/1
  Alpha_Beta_V/1 -> V/1, Beta/1
  Add/1 -> CY/1
  Product1/1 -> Add/5
  Product3/1 -> Add/4

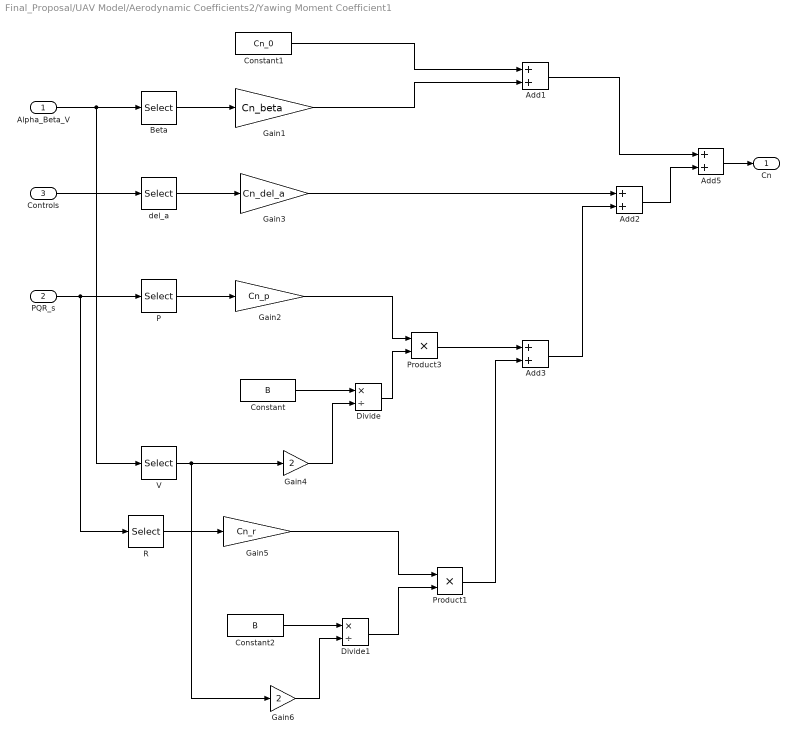
== system Final_Proposal/UAV Model/Aerodynamic Coefficients2/Yawing Moment Coefficient1 ==
  Alpha_Beta_V : Inport
  PQR_s : Inport  Port=2
  Controls : Inport  Port=3
  Add{1..3,5} (4 alike) : Sum
  Beta : Selector  InputPortWidth=3  IndexOptions=Index vector (dialog)  Indices=[2]  OutputSizes=1
  Constant : Constant  Value=B
  Constant1 : Constant  Value=Cn_0
  Constant2 : Constant  Value=B
  Divide : Product  Inputs=*/
  Divide1 : Product  Inputs=*/
  Gain1 : Gain  Gain=Cn_beta
  Gain2 : Gain  Gain=Cn_p
  Gain3 : Gain  Gain=Cn_del_a
  Gain4 : Gain  Gain=2
  Gain5 : Gain  Gain=Cn_r
  Gain6 : Gain  Gain=2
  P : Selector  InputPortWidth=3  IndexOptions=Index vector (dialog)  Indices=[1]  OutputSizes=1
  Product1 : Product
  Product3 : Product
  R : Selector  InputPortWidth=3  IndexOptions=Index vector (dialog)  Indices=[3]  OutputSizes=1
  V : Selector  InputPortWidth=3  IndexOptions=Index vector (dialog)  Indices=[3]  OutputSizes=1
  del_a : Selector  InputPortWidth=3  IndexOptions=Index vector (dialog)  Indices=[2]  OutputSizes=1
  Cn : Outport  VectorParamsAs1DForOutWhenUnconnected=off
  wires:
  R/1 -> Gain5/1
  Divide1/1 -> Product1/2
  Constant2/1 -> Divide1/1
  Gain6/1 -> Divide1/2
  Gain5/1 -> Product1/1
  V/1 -> Gain6/1, Gain4/1
  Add2/1 -> Add5/2
  Gain1/1 -> Add1/2
  Constant/1 -> Divide/1
  PQR_s/1 -> R/1, P/1
  Gain4/1 -> Divide/2
  Gain3/1 -> Add2/1
  Divide/1 -> Product3/2
  Add1/1 -> Add5/1
  Gain2/1 -> Product3/1
  Constant1/1 -> Add1/1
  Alpha_Beta_V/1 -> V/1, Beta/1
  Beta/1 -> Gain1/1
  P/1 -> Gain2/1
  Product3/1 -> Add3/1
  Product1/1 -> Add3/2
  del_a/1 -> Gain3/1
  Controls/1 -> del_a/1
  Add5/1 -> Cn/1
  Add3/1 -> Add2/2

== system Final_Proposal/UAV Model/Propulsive Force and Moment/N(RPS) ==
  Controls : Inport
  Constant1 : Constant  Value=60
  Constant2 : Constant  Value=7000
  Divide : Product  Inputs=*/
  Gain2 : Gain  Gain=20000
  Sum : Sum  Inputs=|++
  del_th : Selector  InputPortWidth=3  IndexOptions=Index vector (dialog)  Indices=[3]  OutputSizes=1
  Out1 : Outport
  wires:
  Controls/1 -> del_th/1
  Sum/1 -> Divide/1
  Divide/1 -> Out1/1
  Gain2/1 -> Sum/2
  Constant1/1 -> Divide/2
  del_th/1 -> Gain2/1
  Constant2/1 -> Sum/1

== system Final_Proposal/UAV Model/Subsystem1/Altitude - ISA Analysis ==
  h : Inport
  ISA Atmosphere Model : aerolibatmos2/ISA Atmosphere Model  useExtended=off  action=Warning  custom=off  viscosityOut=off  g=9.80665  gamma=1.4  R=287.0531  L=0.0065  h_trop=11000  h_strat=20000  rho0=1.225  P0=101325  T0=288.15  h0=0  S=110.4  Tref=273.15  muref=1.716e-5
  Terminator : Terminator
  Terminator1 : Terminator
  Terminator2 : Terminator
  Rho : Outport
  wires:
  ISA Atmosphere Model/4 -> Rho/1  "Rho"
  ISA Atmosphere Model/1 -> Terminator/1
  ISA Atmosphere Model/2 -> Terminator2/1  "a"
  ISA Atmosphere Model/3 -> Terminator1/1
  h/1 -> ISA Atmosphere Model/1

== system Final_Proposal/UAV Model/Total Force & Moment/Subsystem ==
  cE_B : Inport
  Constant : Constant  Value=0
  Constant1 : Constant  Value=Mass
  "Gravity vector in body frame " : Product  Multiplication=Matrix(*)  InputSameDT=on  SaturateOnIntegerOverflow=on  OutDataTypeStr=Inherit: Same as first input
  Mux1 : Mux  Inputs=3
  g : Gain  Gain=UNIT_GRAV
  Gravity : Outport  VectorParamsAs1DForOutWhenUnconnected=off
  wires:
  cE_B/1 -> "Gravity vector in body frame "/1
  "Gravity vector in body frame "/1 -> Gravity/1
  Constant/1 -> Mux1/1, Mux1/2
  g/1 -> Mux1/3
  Mux1/1 -> "Gravity vector in body frame "/2
  Constant1/1 -> g/1

== system Final_Proposal/UAV Model/Total Force & Moment/Total Force & Moment ==
  note: Total Force and Moment
  F_aero : Inport  PortDimensions=3
  M_aero : Inport  Port=2  PortDimensions=3
  F_gravity : Inport  Port=3  PortDimensions=3
  F_prop : Inport  Port=4  PortDimensions=3
  M_prop : Inport  Port=5  PortDimensions=3
  Total Force : Sum  Inputs=+++  InputSameDT=on  SaturateOnIntegerOverflow=on  OutDataTypeStr=Inherit: Same as first input
  Total Moment : Sum  InputSameDT=on  SaturateOnIntegerOverflow=on  OutDataTypeStr=Inherit: Same as first input
  F_cg : Outport  VectorParamsAs1DForOutWhenUnconnected=off
  M_cg : Outport  Port=2  VectorParamsAs1DForOutWhenUnconnected=off
  wires:
  F_gravity/1 -> Total Force/3
  Total Moment/1 -> M_cg/1
  F_prop/1 -> Total Force/2
  F_aero/1 -> Total Force/1
  Total Force/1 -> F_cg/1
  M_aero/1 -> Total Moment/1
  M_prop/1 -> Total Moment/2
